simulink model "freefall"  (R2014a)
settings: Solver=ode45  StartTime=0.0  StopTime=10.0  RelTol=1e-3
settings Model: Creator=eruffaldi  LastModifiedBy=eruffaldi

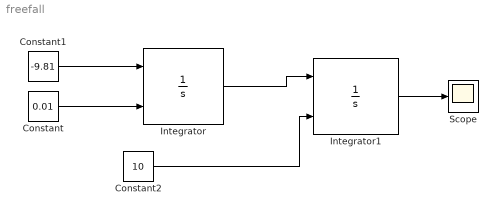
== system freefall ==
  Constant : Constant  Value=0.01
  Constant1 : Constant  Value=-9.81
  Constant2 : Constant  Value=10
  Integrator : Integrator  InitialConditionSource=external
  Integrator1 : Integrator  InitialConditionSource=external  LimitOutput=on  LowerSaturationLimit=0
  Scope : Scope
  wires:
  Constant/1 -> Integrator/2
  Constant1/1 -> Integrator/1
  Integrator/1 -> Integrator1/1
  Integrator1/1 -> Scope/1
  Constant2/1 -> Integrator1/2
